simulink model "RHSmtlfuncInteg_dgl"  (R2021a)
settings: Solver=ode1  StartTime=0.0  StopTime=20  FixedStep=0.001  RelTol=1e-3  EnableMultiTasking=on
PostLoadFcn:
  | , if any(exist('dsrtsu_mdlpostloadfcn', 'file') == [2, 3, 6]), try dsrtsu_mdlpostloadfcn('Execute', bdroot); catch fprintf('Error in PostLoadFcn (dsrtsu_mdlpostloadfcn) for model "%s":\n %s\n', bdroot, lasterr); end, end,
undefined symbols (not defined in the file or in its folder): mygain
settings Model: DSRTSU_INTERNAL_RTI_VER=550  DSRTSU_INTERNAL_RTI_TYPE=rti1202  DSRTSU_INTERNAL_RTIFPGA=150  RTICANMMDATA=struct('GeneralSetupData',struct('modelroot','C:\Users\nitr\Documents\PURfolien\2020\IMC\matlab','generalsettings',struct('filesettings',struct('destfolder',struct('Name','RTICANMM_FILES','Check',1),'buildfolder',struct('Name','.','Check',1),'AbsDestfolder',struct('Name','C:\Users\nitr\Documents\PURfolien\2020\IMC\matlab\RTICANMM_FILES'),'AbsBuildfolder',struct('Name','C:\Users\nitr\Documents\PURfolien\2020\IMC\matlab'))),'options',struct('addpaths',1,'rmpaths',1,'addtrcexclusion',true,'cannavigator',struct('checkmonitoring',0),'show_usrtrc',0,'use_usrtrc',0),'advanced',struct('options',ones(1,100)),'MPSetup',{{}},'RTI',struct('Type','RTI1005','Ver','7.13','Date','02-Nov-2019'),'modelname','RHSmtlfuncInteg_dgl','block','RHSmtlfuncInteg_dgl'))  Creator=nitr  LastModifiedBy=nitr
settings SolverCC: AlgebraicLoopSolver=TrustRegion
settings DataIOCC: LimitDataPoints=on  SaveFormat=Array  SignalLoggingSaveFormat=ModelDataLogs  ReturnWorkspaceOutputs=off
settings OptimizationCC: BlockReduction=off  OptimizeBlockIOStorage=off  BufferReuse=off  GlobalBufferReuse=off  ExpressionFolding=off  ExpressionDepthLimit=2147483647  LocalBlockOutputs=off  LifeSpan=inf  OptimizeDataStoreBuffers=off  BusAssignmentInplaceUpdate=off
settings DebuggingCC: UnderspecifiedInitializationDetection=Classic  MergeDetectMultiDrivingBlocksExec=none  SolverPrmCheckMsg=warning  FcnCallInpInsideContextMsg=warning  StateNameClashWarn=warning  SFUnexpectedBacktrackingDiag=warning  SFNoUnconditionalDefaultTransitionDiag=warning  SFExecutionAtInitializationDiag=none  SFMachineParentedDataDiag=warning  ArithmeticOperatorsInVariantConditions=warning
settings HardwareCC: ProdBitPerPointer=32  ProdBitPerSizeT=32  ProdBitPerPtrDiffT=32  ProdLargestAtomicInteger=Integer  ProdEndianess=BigEndian  ProdWordSize=32  ProdHWDeviceType=Custom Processor->Custom  TargetIntDivRoundTo=Zero  TargetEndianess=BigEndian  TargetHWDeviceType=Custom Processor->Custom
settings ModelReferenceCC: PropagateSignalLabelsOutOfModel=off
settings SFSimCC: SimUseLocalCustomCode=off  MATLABDynamicMemAlloc=off  CustomCodeUndefinedFunction=UseInterfaceOnly
settings RTWCC: Description=dSPACE DS1005 Hardware Platform  SystemTargetFile=rti1005.tlc  MakeCommand=make_rti  TemplateMakefile=rti1005.tmf  RTWUseLocalCustomCode=off
settings CodeAppCC: StateflowObjectComments=on
settings STFCustomTargetCC: ParMdlRefBuildCompliant=on  MatFileLogging=on  GRTInterface=off  UseToolchainInfoCompliant=off  SystemTargetFile=rti1005.tlc
settings GRTTargetCC: TargetLangStandard=C89/C90 (ANSI)  CompOptLevelCompliant=off  ConcurrentExecutionCompliant=off  CombineOutputUpdateFcns=off  CPPClassGenCompliant=off  UseToolchainInfoCompliant=off  ExtModeMexFile=noextcomm
settings ConfigComp: CovMetricSettings=dw  CovSaveCumulativeToWorkspaceVar=on  CovSaveSingleToWorkspaceVar=on  CovExternalEMLEnable=off  CovSFcnEnable=off

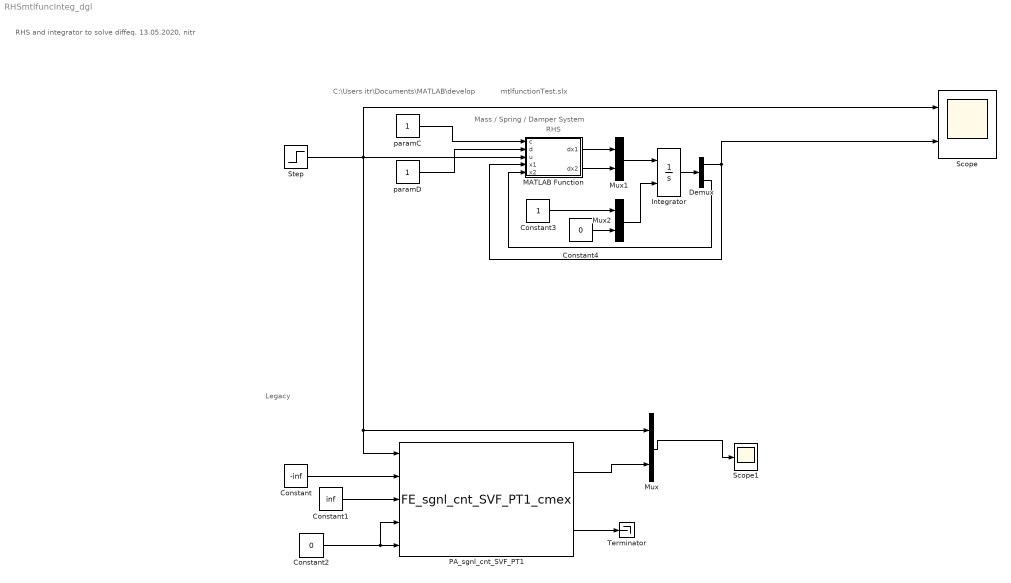
== system RHSmtlfuncInteg_dgl ==
  note: Legacy
  note: Mass / Spring / Damper System
  note: RHS
  note: RHS and integrator to solve diffeq.
      |
      | 13.05.2020, nitr
  note: mtlfunctionTest.slx
  note: C:\Users\nitr\Documents\MATLAB\develop
  Constant : Constant  Value=-inf
  Constant1 : Constant  Value=inf
  Constant2 : Constant  Value=0
  Constant3 : Constant
  Constant4 : Constant  Value=0
  Demux : Demux  Outputs=2
  Integrator : Integrator  InitialConditionSource=external
  MATLAB Function : MATLAB Function  TreatAsAtomicUnit=on
  Mux : Mux  Inputs=2
  Mux1 : Mux  Inputs=2
  Mux2 : Mux  Inputs=2
  PA_sgnl_cnt_SVF_PT1 : S-Function  Tag=PA_sgnl_cnt_SVF_PT1  FunctionName=FE_sgnl_cnt_SVF_PT1_cmex  Parameters=mg % tau*mygain  SFunctionDeploymentMode=off  EnableBusSupport=off  mask(FE_sgnl_cnt_SVF_PT1){tau=1}
      mask prompts: tau "Time constant "tau" in s (>0)"
      mask help:
      | Models the following transfer function:
      |
      | G(s)=Y(s)/U(s)=1/(tau*s +1)
      |
      | The time constant "tau" is a masked block parameter.
      | -----------------------------------------------------------------------------------------
      |
      | Outputs:
      | y
      |
      | dy = dy/dt
      | -----------------------------------------------------------------------------------------
      |
      | Inputs:
      | u
      |
      | dymin: Is the minimum saturation limit for output dy.  Output dy cannot go any lower than dymin.
      |
      | dymax: Is the maximum saturation limit for output dy.  Output dy cannot go any higher than dymin.
      |
      | reset: If this value is not equal to zero all outputs bar the derivative of the highest order will be reset to the start values.
      |
      | y0: Start value for output y-> y(t=0) = y0.
      | -----------------------------------------------------------------------------------------
      |
      | Press "Help" for more information (or Alt + H).
      mask init:
      | mg = tau*.5;
      mask Help: eval(['run(strcat(''',getenv('pasl_simulink'),''',''\documentation\tools\HelpForPaslElements.m''))']);
      mask Display:
      | image(imread('PA_sgnl_cnt_SVF.png'));
      | text(0.25,0.95,'SVF PT1');
      | port_label('output', 1, 'y');
      | port_label('output',2,'dy');
      | port_label('input', 1, 'u');
      | port_label('input', 2, 'dymin');
      | port_label('input', 3, 'dymax');
      | port_label('input', 4, 'reset');
      | port_label('input', 5, 'y0');
  Scope : Scope  NumInputPorts=2
  Scope1 : Scope
  Step : Step  Time=10  SampleTime=0
  Terminator : Terminator
  paramC : Constant
  paramD : Constant
  wires:
  Step/1 -> Scope/1, MATLAB Function/3(u), PA_sgnl_cnt_SVF_PT1/1, Mux/1
  PA_sgnl_cnt_SVF_PT1/1 -> Mux/2
  Mux/1 -> Scope1/1
  Constant/1 -> PA_sgnl_cnt_SVF_PT1/2
  Constant1/1 -> PA_sgnl_cnt_SVF_PT1/3
  Constant2/1 -> PA_sgnl_cnt_SVF_PT1/4, PA_sgnl_cnt_SVF_PT1/5
  PA_sgnl_cnt_SVF_PT1/2 -> Terminator/1
  MATLAB Function/1(dx1) -> Mux1/1
  MATLAB Function/2(dx2) -> Mux1/2
  Mux1/1 -> Integrator/1
  Constant3/1 -> Mux2/1
  Constant4/1 -> Mux2/2
  Mux2/1 -> Integrator/2
  Integrator/1 -> Demux/1
  Demux/1 -> MATLAB Function/4(x1), Scope/2
  Demux/2 -> MATLAB Function/5(x2)
  paramC/1 -> MATLAB Function/1(c)
  paramD/1 -> MATLAB Function/2(d)

== matlab function RHSmtlfuncInteg_dgl/MATLAB Function ==
  data: c input; d input; u input; dx1 output; x1 input; x2 input; dx2 output
function [dx1, dx2] = fcn(c,d,u,x1,x2)
%#codegen

% %% Erstellen des Vorfilters
% lambda_FF = -3;
% Aff = [0 1 0;
% 0 0 1;
% lambda_FF^3 -3*lambda_FF^2 3*lambda_FF];
% bff = [0; 0; -lambda_FF^3];
% cff = [1 0 0;
% 0 1 0;
% 0 0 1;
% lambda_FF^3 -3*lambda_FF^2 3*lambda_FF];
% dff = [0;0;0;-lambda_FF^3];
% % F = ss(Aff,bff,cff,dff);

dx1= x2;
dx2=-c*x2 - d*x1 +u;
